simulink model "PMSM"  (R2024a)
settings: Solver=ode23tb  StartTime=0.0  StopTime=10.0  MaxStep=1e-4  RelTol=1e-4
values from neighbouring files (symbols this model uses):
  B = 4.047e-5    (= 4.047e-05)    [pmsm_script.m]
  flux = 0.1848    [pmsm_script.m]
  J = 0.0001051    [pmsm_script.m]
  Ld = 0.014    [pmsm_script.m]
  Lq = 0.014    [pmsm_script.m]
  P = 2    [pmsm_script.m]
  Rs = 4.765    [pmsm_script.m]
  Vm = 100    [pmsm_script.m]
settings Model: Creator=Saswata Mahato  LastModifiedBy=Saswata Mahato

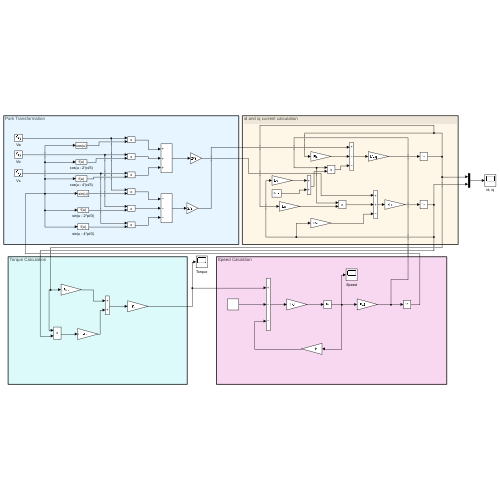
[thumbnail: Simulink's stored preview of the top-level diagram]
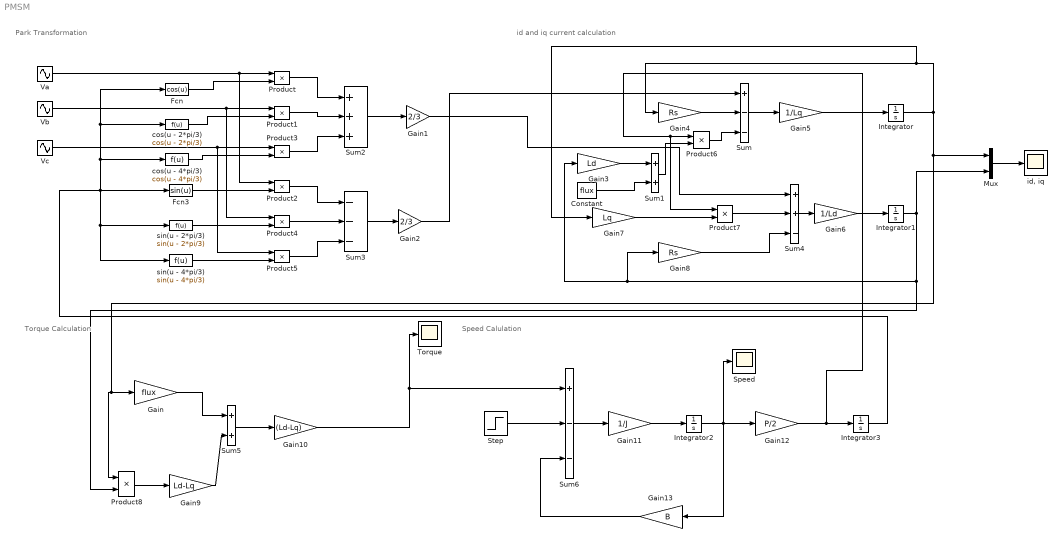
== system PMSM ==
  note: Speed Calulation
  note: Torque Calculation
  note: id and iq current calculation
  note: Park Transformation
  Constant : Constant  Value=flux
  Fcn : Fcn  Expr=cos(u)
  Fcn3 : Fcn  Expr=sin(u)
  Gain : Gain  Gain=flux
  Gain1 : Gain  Gain=2/3
  Gain10 : Gain  Gain=(Ld-Lq)
  Gain11 : Gain  Gain=1/J
  Gain12 : Gain  Gain=P/2
  Gain13 : Gain  Gain=B
  Gain2 : Gain  Gain=2/3
  Gain3 : Gain  Gain=Ld
  Gain4 : Gain  Gain=Rs
  Gain5 : Gain  Gain=1/Lq
  Gain6 : Gain  Gain=1/Ld
  Gain7 : Gain  Gain=Lq
  Gain8 : Gain  Gain=Rs
  Gain9 : Gain  Gain=Ld-Lq
  Integrator{,1..3} (4 alike) : Integrator
  Mux : Mux  Inputs=2
  Product{,1..8} (9 alike) : Product
  Speed : Scope
  Step : Step  Time=0.5  After=1.7  SampleTime=0
  Sum : Sum  Inputs=+--
  Sum1 : Sum
  Sum2 : Sum  Inputs=+++
  Sum3 : Sum  Inputs=---
  Sum4 : Sum  Inputs=++-
  Sum5 : Sum
  Sum6 : Sum  Inputs=+--
  Torque : Scope
  Va : Sin  Amplitude=Vm  Frequency=2*pi*50  SampleTime=0
  Vb : Sin  Amplitude=Vm  Frequency=2*pi*50  Phase=-2*pi/3  SampleTime=0
  Vc : Sin  Amplitude=Vm  Frequency=2*pi*50  Phase=2*pi/3  SampleTime=0
  cos(u - 2*pi/3) : Fcn  Expr=cos(u - 2*pi/3)
  cos(u - 4*pi/3) : Fcn  Expr=cos(u - 4*pi/3)
  "id, iq" : Scope
  sin(u - 2*pi/3) : Fcn  Expr=sin(u - 2*pi/3)
  sin(u - 4*pi/3) : Fcn  Expr=sin(u - 4*pi/3)
  wires:
  Vc/1 -> Product5/1, Product3/1
  sin(u - 4*pi/3)/1 -> Product5/2
  sin(u - 2*pi/3)/1 -> Product4/2
  Fcn3/1 -> Product2/2
  cos(u - 2*pi/3)/1 -> Product1/2
  Fcn/1 -> Product/2
  Product1/1 -> Sum2/2
  Product/1 -> Sum2/1
  Product3/1 -> Sum2/3
  Product2/1 -> Sum3/1
  Product4/1 -> Sum3/2
  Product5/1 -> Sum3/3
  Sum2/1 -> Gain1/1
  Sum3/1 -> Gain2/1
  cos(u - 4*pi/3)/1 -> Product3/2
  Gain4/1 -> Sum/2
  Sum/1 -> Gain5/1
  Product6/1 -> Sum/3
  Gain3/1 -> Sum1/1
  Sum1/1 -> Product6/2
  Product7/1 -> Sum4/2
  Gain8/1 -> Sum4/3
  Sum4/1 -> Gain6/1
  Gain7/1 -> Product7/2
  Gain5/1 -> Integrator/1
  Gain6/1 -> Integrator1/1
  Integrator1/1 -> Mux/2, Product8/2, Gain8/1, Gain3/1
  Constant/1 -> Sum1/2
  Product8/1 -> Gain9/1
  Gain9/1 -> Sum5/2
  Gain/1 -> Sum5/1
  Sum5/1 -> Gain10/1
  Sum6/1 -> Gain11/1
  Gain11/1 -> Integrator2/1
  Integrator2/1 -> Speed/1, Gain13/1, Gain12/1
  Gain13/1 -> Sum6/3
  Va/1 -> Product2/1, Product/1
  Vb/1 -> Product4/1, Product1/1
  Gain2/1 -> Sum/1
  Gain1/1 -> Sum4/1
  Integrator/1 -> Product8/1, Gain/1, Mux/1, Gain4/1, Gain7/1
  Gain10/1 -> Torque/1, Sum6/1
  Step/1 -> Sum6/2
  Gain12/1 -> Integrator3/1, Product6/1, Product7/1
  Mux/1 -> "id, iq"/1
  Integrator3/1 -> sin(u - 2*pi/3)/1, sin(u - 4*pi/3)/1, Fcn/1, cos(u - 2*pi/3)/1, cos(u - 4*pi/3)/1, Fcn3/1
